simulink model "SoftStarterACVV"  (R2016a)
settings: Solver=ode45  StartTime=0.0  StopTime=5  RelTol=1e-3
undefined symbols (not defined in the file): D1, lagging, pulse
libraries: spsThyristorLib x6, spsACVoltageSourceLib x3, spsThreePhaseVIMeasurementLib x2, spsAsynchronousMachineSIUnitsLib x1, spsGroundLib x1, spsPLL3phLib x1, spsPulseGeneratorThyristor12PulseLib x1, spspowerguiLib x1
settings Model: Creator=khaled18  LastModifiedBy=IBRAHEM SHQAIR
settings DataIOCC: LimitDataPoints=on  SaveFormat=Array
settings DebuggingCC: SolverPrmCheckMsg=warning
settings HardwareCC: ProdBitPerPointer=32  ProdLargestAtomicFloat=None  ProdIntDivRoundTo=Undefined  ProdEndianess=Unspecified  ProdWordSize=32  ProdHWDeviceType=32-bit Generic
settings ModelReferenceCC: PropagateSignalLabelsOutOfModel=off
settings ConfigComp: CovSFcnEnable=off
settings SimscapeCC: SimscapeNormalizeSystem=off

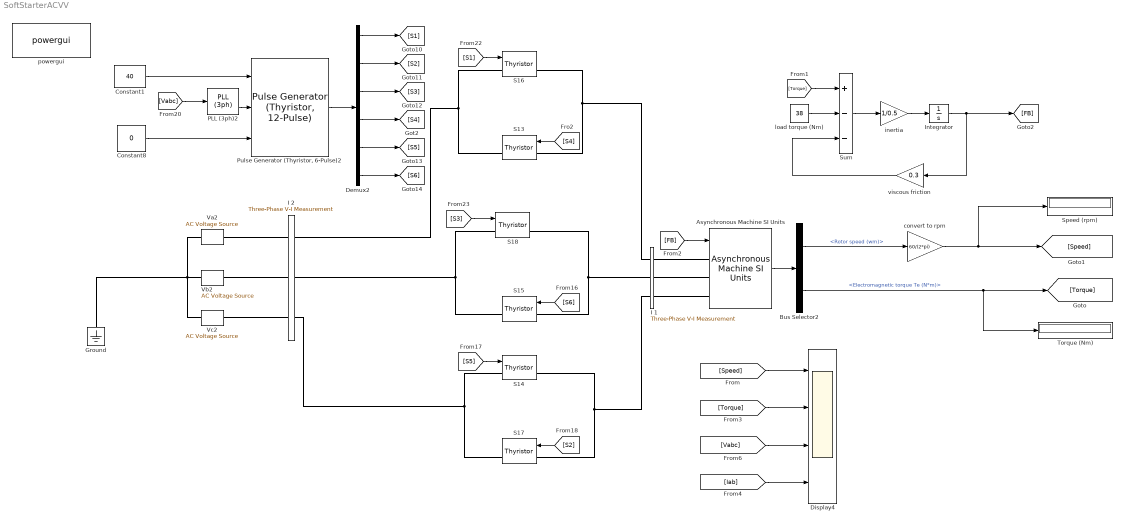
== system SoftStarterACVV ==
  Asynchronous Machine SI Units : spsAsynchronousMachineSIUnitsLib/Asynchronous Machine SI Units  RotorType=Squirrel-cage  PresetModel="01:  5 HP   460 V 60Hz 1750 RPM"  MechanicalLoad=Speed w  ShowDetailedParameters=on  ReferenceFrame=Rotor  Units=SI  MeasurementBus=off  NominalParameters=[3730 460 60]  VoltageRatio=1  Stator=[1.115 0.005974]  Rotor=[1.083 0.005974]  Cage1=[ 0.022 0.226/377]  Cage2=[ 0.022 0.226/377]  Lm=0.2037  Mechanical=[0.02 0.005752 2]  PolePairs=2  InitialConditions=[1 0 0 0 0 0 0 0]  SimulateSaturation=off  Saturation=[14.03593122, 27.81365428, 53.79336849, 72.68890987, 97.98006896, 148.6815601, 215.7428561, 302.9841135, 428.7778367 ; 230, 322, 414, 460, 506, 552, 598, 644, 690]  LoadFlowParameters=1492000  TsPowergui=0  TsBlock=-1  IterativeModel=Forward Euler  IterativeDiscreteModel=Trapezoidal non iterative  Pmec=0
      settings: AttributesFormatString=\n
  Bus Selector2 : BusSelector  OutputSignals=Mechanical.Rotor speed (wm),Mechanical.Electromagnetic torque Te (N*m)
  Constant1 : Constant  Value=40
  Constant8 : Constant  Value=0
  Demux2 : Demux  Outputs=6
  Display4 : Scope  NumInputPorts=4
  Ground : spsGroundLib/Ground  LConnTagsString=a
  I 1 : spsThreePhaseVIMeasurementLib/Three-Phase V-I Measurement  VoltageMeasurement=phase-to-phase  SetLabelV=on  LabelV=Vabc1  Vpu=off  VpuLL=off  CurrentMeasurement=yes  SetLabelI=on  LabelI=Iabc1  Ipu=off  Pbase=100e6  Vbase=500e3  OutputType=Complex  PhasorSimulation=off  PSBequivalent=0
  I 2 : spsThreePhaseVIMeasurementLib/Three-Phase V-I Measurement  VoltageMeasurement=phase-to-ground  SetLabelV=on  LabelV=Vabc  Vpu=off  VpuLL=off  CurrentMeasurement=yes  SetLabelI=on  LabelI=Iab  Ipu=off  Pbase=100e6  Vbase=500e3  OutputType=Complex  PhasorSimulation=off  PSBequivalent=0
  Integrator : Integrator
  PLL (3ph)2 : spsPLL3phLib/PLL (3ph)  Fmin=45  Par_Init=[0, 50]  ParK=[180, 3200, 1]  TcD=1e-4  MaxRateChangeFreq=12  FilterCutOffFreq=25  Ts=0  AGC=on
  "Pulse Generator (Thyristor, 6-Pulse)2" : spsPulseGeneratorThyristor12PulseLib/Pulse Generator (Thyristor, 12-Pulse)  GenType=6-pulse  Delta=D1 (lagging)  pwidth=50  Double_Pulse=on  Ts=0
  S{13..18} (6 alike) : spsThyristorLib/Thyristor  Ron=0.001  Lon=0  Vf=0.8  IC=0  Rs=500  Cs=250e-9  Measurements=on
  Speed (rpm) : Display
  Sum : Sum  Inputs=+--
  Torque (Nm) : Display
  Va2 : spsACVoltageSourceLib/AC Voltage Source  Amplitude=460  Phase=0  Frequency=50  SampleTime=0  Measurements=None  BusType=swing  Pref=10e3  Qref=0  Qmin=-inf  Qmax=+inf
  Vb2 : spsACVoltageSourceLib/AC Voltage Source  Amplitude=460  Phase=-120  Frequency=50  SampleTime=0  Measurements=None  BusType=swing  Pref=10e3  Qref=0  Qmin=-inf  Qmax=+inf
  Vc2 : spsACVoltageSourceLib/AC Voltage Source  Amplitude=460  Phase=120  Frequency=50  SampleTime=0  Measurements=None  BusType=swing  Pref=10e3  Qref=0  Qmin=-inf  Qmax=+inf
  convert to rpm : Gain  Gain=60/(2*pi)
  inertia : Gain  Gain=1/0.5
  load torque (Nm) : Constant  Value=38
  powergui : spspowerguiLib/powergui  Priority=1  SimulationMode=Discrete  SampleTime=50e-6  frequency=60  Iterations=50  frequencyindice=50  Pbase=100e6  ErrMax=1e-4  UnitsV=kV  UnitsW=MW  buscounter=0  FunctionMessages=off  echomessages=off  EnableUseOfTLC=off  CurrentSourceSwitches=off  DisableSnubberDevices=off  DisableRonSwitches=off  DisableVfSwitches=off  DisplayEquations=off  AutomaticDiscreteSolvers=off  SolverType=Tustin/Backward Euler (TBE)  Interpol=off  ExternalGateDelay=off  methode=off  Ts=100  x0status=blocks  SPID=off  SwTol=0  HookPort=off  NonlinearTolerance=1e-4  nMaxIteration=100  ContinueOnMaxIteration=off  RestoreLinks=warning  ResistiveCurrentMeasurement=off  Frange=[0:2:500]  Ylog=off  Xlog=on  ShowGrid=off  save=off  variable=ZData  structure=0  ZoomFFT=off  StartTime=0.0  cycles=1  DisplayStyle=1  fundamental=60  FreqAxis=off  MaxFrequency=1000  frequencyindicesteady=1  RmsSteady=1  display=off
  viscous friction : Gain  Gain=0.3
  wires:
  [Vabc] -> PLL (3ph)2/1
  Constant8/1 -> "Pulse Generator (Thyristor, 6-Pulse)2"/3
  "Pulse Generator (Thyristor, 6-Pulse)2"/1 -> Demux2/1
  [S4] -> S13/1
  [S5] -> S14/1
  Demux2/4 -> [S4]
  Asynchronous Machine SI Units/1 -> Bus Selector2/1
  [S6] -> S15/1
  Demux2/5 -> [S5]
  Demux2/2 -> [S2]
  Demux2/6 -> [S6]
  PLL (3ph)2/2 -> "Pulse Generator (Thyristor, 6-Pulse)2"/2
  [S1] -> S16/1
  Demux2/1 -> [S1]
  [S3] -> S18/1
  Demux2/3 -> [S3]
  [S2] -> S17/1
  Constant1/1 -> "Pulse Generator (Thyristor, 6-Pulse)2"/1
  Bus Selector2/2 -> Torque (Nm)/1, [Torque]  "<Electromagnetic torque Te (N*m)>"
  Sum/1 -> inertia/1
  inertia/1 -> Integrator/1
  Integrator/1 -> viscous friction/1, [FB]
  Bus Selector2/1 -> convert to rpm/1  "<Rotor speed (wm)>"
  [Torque] -> Sum/1
  load torque (Nm)/1 -> Sum/2
  viscous friction/1 -> Sum/3
  [FB] -> Asynchronous Machine SI Units/1
  convert to rpm/1 -> Speed (rpm)/1, [Speed]
  [Speed] -> Display4/1
  [Torque] -> Display4/2
  [Vabc] -> Display4/3
  [Iab] -> Display4/4
  connections:
  S16/LConn1 -- I 2/RConn1 -- S13/RConn1
  I 2/RConn3 -- S17/RConn1 -- S14/LConn1
  S15/RConn1 -- I 2/RConn2 -- S18/LConn1
  S18/RConn1 -- I 1/LConn2 -- S15/LConn1
  Vc2/LConn1 -- Vb2/LConn1 -- Ground/LConn1 -- Va2/LConn1
  S14/RConn1 -- I 1/LConn3 -- S17/LConn1
  S16/RConn1 -- S13/LConn1 -- I 1/LConn1
  I 2/LConn3 -- Vc2/RConn1
  I 2/LConn2 -- Vb2/RConn1
  I 2/LConn1 -- Va2/RConn1
  I 1/RConn1 -- Asynchronous Machine SI Units/LConn1
  I 1/RConn2 -- Asynchronous Machine SI Units/LConn2
  I 1/RConn3 -- Asynchronous Machine SI Units/LConn3
